simulink model "TuNT54_day2_homework"  (R2017b)
settings: Solver=FixedStepDiscrete  StartTime=0.0  StopTime=10.0  RelTol=1e-3
PreLoadFcn:
  | run("TuNT54_day2.m")
InitFcn:
  | run("TuNT54_day2.m")
values from neighbouring files (symbols this model uses):
  g = 9.8    [TuNT54_day2.m]
  h = 1    [TuNT54_day2.m]
  v0 = 5    [TuNT54_day2.m]
settings Model: Creator=Admin  LastModifiedBy=Admin
settings OptimizationCC: DefaultParameterBehavior=Inlined  UseDivisionForNetSlopeComputation=on  UseFloatMulNetSlope=on  InlineInvariantSignals=on  PassReuseOutputArgsAs=Individual arguments  ZeroExternalMemoryAtStartup=off  ZeroInternalMemoryAtStartup=off  NoFixptDivByZeroProtection=on  EfficientFloat2IntCast=on  LifeSpan=1
settings DebuggingCC: ParameterTunabilityLossMsg=error
settings HardwareCC: ProdLongLongMode=on
settings SFSimCC: MATLABDynamicMemAlloc=off
settings RTWCC: SystemTargetFile=ert.tlc  TemplateMakefile=ert_default_tmf  GenerateReport=on  IncludeHyperlinkInReport=on  LaunchReport=on  GenerateTraceInfo=on  GenerateTraceReport=on  GenerateTraceReportSl=on  GenerateTraceReportSf=on  GenerateTraceReportEml=on  GenerateCodeMetricsReport=on
settings CodeAppCC: ForceParamTrailComments=on  IgnoreCustomStorageClasses=off  OperatorAnnotations=on  SimulinkDataObjDesc=on  SFDataObjDesc=on  CustomSymbolStrGlobalVar=rt$N$M  CustomSymbolStrType=$N$M  CustomSymbolStrFcn=$N$M$F  CustomSymbolStrMacro=$N$M  InsertBlockDesc=on
settings ERTTargetCC: TargetLangStandard=C99 (ISO)  GenerateSampleERTMain=on  IncludeMdlTerminateFcn=off  CombineSignalStateStructs=on  SuppressErrorStatus=on  SupportAbsoluteTime=off  SupportComplex=off  InlinedParameterPlacement=NonHierarchical  ERTCustomFileTemplate=example_file_process.tlc  ERTFilePackagingFormat=CompactWithDataFile

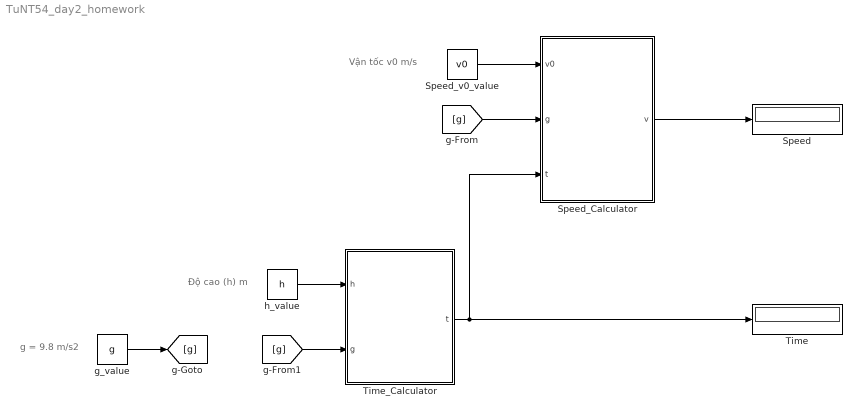
== system TuNT54_day2_homework ==
  note: Độ cao (h) m
  note: g = 9.8 m/s2
  note: Vận tốc v0 m/s
  Speed : Display
  Speed_Calculator : Subsystem
  Speed_v0_value : Constant  Value=v0  OutDataTypeStr=double
  Time : Display
  Time_Calculator : Subsystem
  g_value : Constant  Value=g  OutDataTypeStr=double
  h_value : Constant  Value=h  OutDataTypeStr=double
  wires:
  g_value/1 -> [g]
  Speed_v0_value/1 -> Speed_Calculator/1(v0)
  [g] -> Speed_Calculator/2(g)
  Speed_Calculator/1(v) -> Speed/1
  h_value/1 -> Time_Calculator/1(h)
  [g] -> Time_Calculator/2(g)
  Time_Calculator/1(t) -> Speed_Calculator/3(t), Time/1

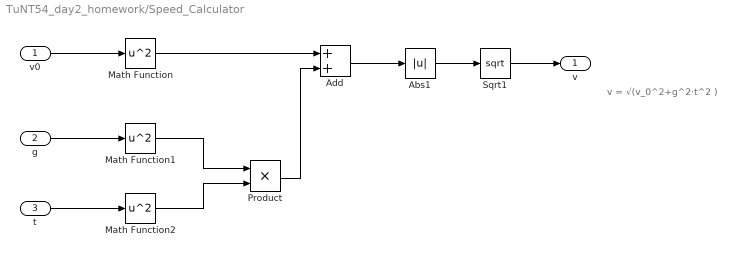
== system TuNT54_day2_homework/Speed_Calculator ==
  note: v = √(v_0^2+g^2⋅t^2 )
  v0 : Inport
  g : Inport  Port=2
  t : Inport  Port=3
  Abs1 : Abs
  Add : Sum
  Math Function : Math  Operator=square  SaturateOnIntegerOverflow=on
  Math Function1 : Math  Operator=square  SaturateOnIntegerOverflow=on
  Math Function2 : Math  Operator=square  SaturateOnIntegerOverflow=on
  Product : Product
  Sqrt1 : Sqrt  SaturateOnIntegerOverflow=on
  v : Outport
  wires:
  Math Function/1 -> Add/1
  g/1 -> Math Function1/1
  Math Function1/1 -> Product/1
  v0/1 -> Math Function/1
  Product/1 -> Add/2
  Abs1/1 -> Sqrt1/1
  Add/1 -> Abs1/1
  Sqrt1/1 -> v/1
  Math Function2/1 -> Product/2
  t/1 -> Math Function2/1

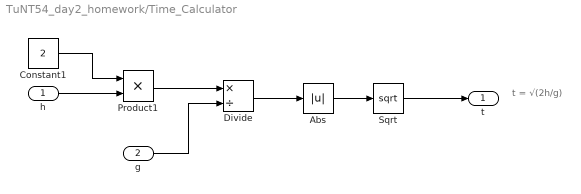
== system TuNT54_day2_homework/Time_Calculator ==
  note: t = √(2h/g)
  h : Inport
  g : Inport  Port=2
  Abs : Abs
  Constant1 : Constant  Value=2
  Divide : Product  Inputs=*/
  Product1 : Product
  Sqrt : Sqrt  SaturateOnIntegerOverflow=on
  t : Outport
  wires:
  g/1 -> Divide/2
  Abs/1 -> Sqrt/1
  Sqrt/1 -> t/1
  Product1/1 -> Divide/1
  h/1 -> Product1/2
  Divide/1 -> Abs/1
  Constant1/1 -> Product1/1
